simulink model "ESTS_FRIC_test"  (R2023b)
settings: Solver=VariableStepAuto  StartTime=0.0  StopTime=10.0  RelTol=1e-3
libraries: ESTS_FRIC x1, simulink x1
settings Model: Creator=blatak  LastModifiedBy=blatak

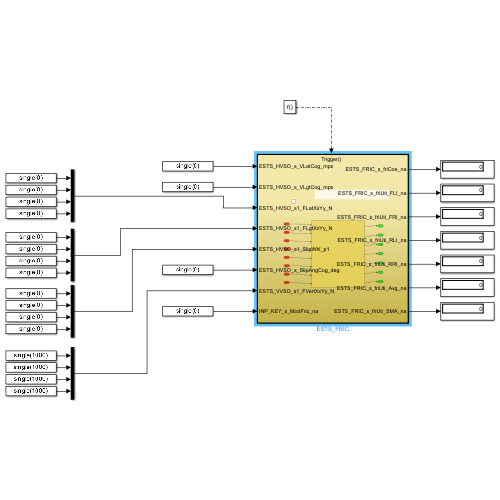
[thumbnail: Simulink's stored preview of the top-level diagram]
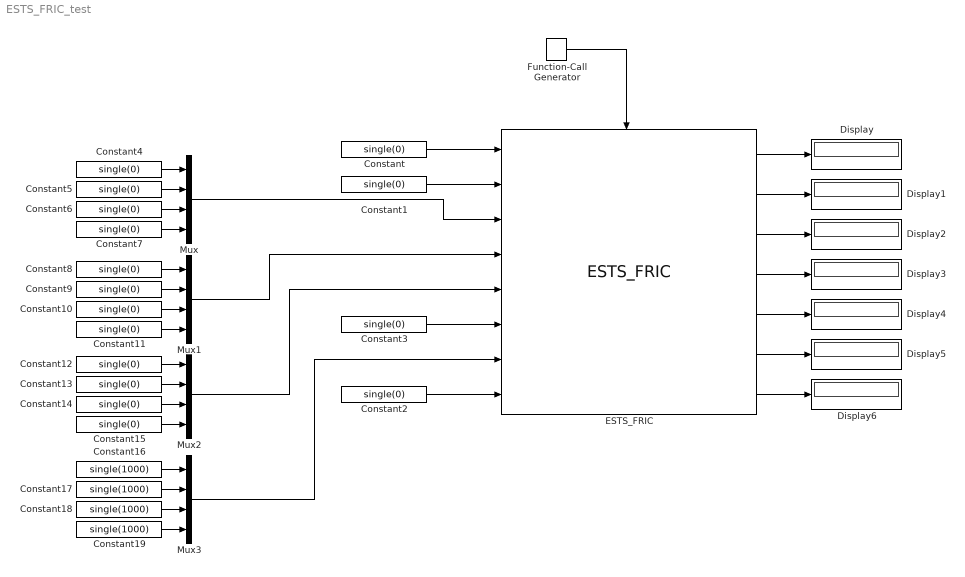
== system ESTS_FRIC_test ==
  Constant{,1..15} (16 alike) : Constant  Value=single(0)
  Constant{16..19} (4 alike) : Constant  Value=single(1000)
  Display{,1..6} (7 alike) : Display
  ESTS_FRIC : ESTS_FRIC/ESTS_FRIC  SystemSampleTime=-1  VariantActivationTime=update diagram  AllowFlexibleInterface=on  Latency=0  AutoFrameSizeCalculation=off
  Function-Call Generator : simulink/Ports & Subsystems/Function-Call Generator  sample_time=0.01  numberOfIterations=1  DisallowWideOutput=off
  Mux{,1..3} (4 alike) : Mux
  wires:
  Function-Call Generator/1 -> ESTS_FRIC/Trigger
  Constant/1 -> ESTS_FRIC/1
  Constant1/1 -> ESTS_FRIC/2
  Constant2/1 -> ESTS_FRIC/8
  Constant3/1 -> ESTS_FRIC/6
  Constant4/1 -> Mux/1
  Constant5/1 -> Mux/2
  Constant7/1 -> Mux/4
  Constant6/1 -> Mux/3
  Constant11/1 -> Mux1/4
  Constant9/1 -> Mux1/2
  Constant8/1 -> Mux1/1
  Constant10/1 -> Mux1/3
  Constant15/1 -> Mux2/4
  Constant13/1 -> Mux2/2
  Constant12/1 -> Mux2/1
  Constant14/1 -> Mux2/3
  Mux/1 -> ESTS_FRIC/3
  Mux1/1 -> ESTS_FRIC/4
  Mux2/1 -> ESTS_FRIC/5
  Constant19/1 -> Mux3/4
  Constant17/1 -> Mux3/2
  Constant16/1 -> Mux3/1
  Constant18/1 -> Mux3/3
  Mux3/1 -> ESTS_FRIC/7
  ESTS_FRIC/1 -> Display/1
  ESTS_FRIC/2 -> Display1/1
  ESTS_FRIC/3 -> Display2/1
  ESTS_FRIC/4 -> Display3/1
  ESTS_FRIC/5 -> Display4/1
  ESTS_FRIC/6 -> Display5/1
  ESTS_FRIC/7 -> Display6/1
